simulink model "Integrate_SubMode_Motor_2021b"  (R2021b)
settings: Solver=FixedStepAuto  StartTime=0.0  StopTime=inf  FixedStep=Ts  RelTol=1e-3  EnableMultiTasking=on
values from neighbouring files (symbols this model uses):
  den_Gd = Gd.Den{:}    [para.m]
  Ki = 0.003    [para.m]
  Kp = 0.0001    [para.m]
  num_Gd = Gd.Num{:}    [para.m]
  rpm_scale = 1/12/4*60    (= 1.25)    [para.m]
  Ts = 0.01    [para.m]
  Wref = 4000    [para.m]
undefined symbols (not defined in the file or in its folder): ADC_MAX, cycle_per_rotate, ENCODER_MAX, Kd, RPM_MAX, sec_per_minute
libraries: arduinolib x17, simulink x4, arduinosensorlib x4, slpidlib x1
settings Model: SimulationMode=external  ExtModeTrigDuration=2  Creator=user  LastModifiedBy=user
settings SolverCC: AutoInsertRateTranBlk=on
settings OptimizationCC: EnhancedBackFolding=on  PassReuseOutputArgsAs=Individual arguments  ZeroExternalMemoryAtStartup=off  ZeroInternalMemoryAtStartup=off  MaxStackSize=64  OptimizeBlockOrder=speed  DifferentSizesBufferReuse=on  OptimizationCustomize=off  EfficientTunableParamExpr=on
settings DebuggingCC: ParameterTunabilityLossMsg=error
settings HardwareCC: ProdBitPerInt=16  ProdBitPerPointer=16  ProdBitPerSizeT=16  ProdBitPerPtrDiffT=16  ProdLargestAtomicFloat=None  ProdWordSize=8  ProdHWDeviceType=Atmel->AVR
settings SFSimCC: MATLABDynamicMemAlloc=off
settings RTWCC: Description=Embedded Coder  SystemTargetFile=ert.tlc  HardwareBoard=Arduino Mega 2560  TemplateMakefile=ert_default_tmf  Toolchain=Arduino AVR  BuildConfiguration=Faster Runs
settings CodeAppCC: ForceParamTrailComments=on  IgnoreCustomStorageClasses=off  OperatorAnnotations=on  SimulinkDataObjDesc=on  SFDataObjDesc=on  InsertBlockDesc=on
settings ERTTargetCC: SupportContinuousTime=on  SupportVariableSizeSignals=on  ExtMode=on  ExtModeStaticAlloc=on  ExtModeStaticAllocSize=2048  ExtModeMexArgs='' 0 17725

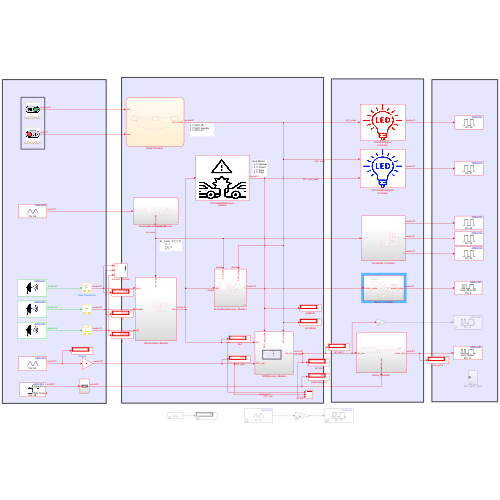
[thumbnail: Simulink's stored preview of the top-level diagram]
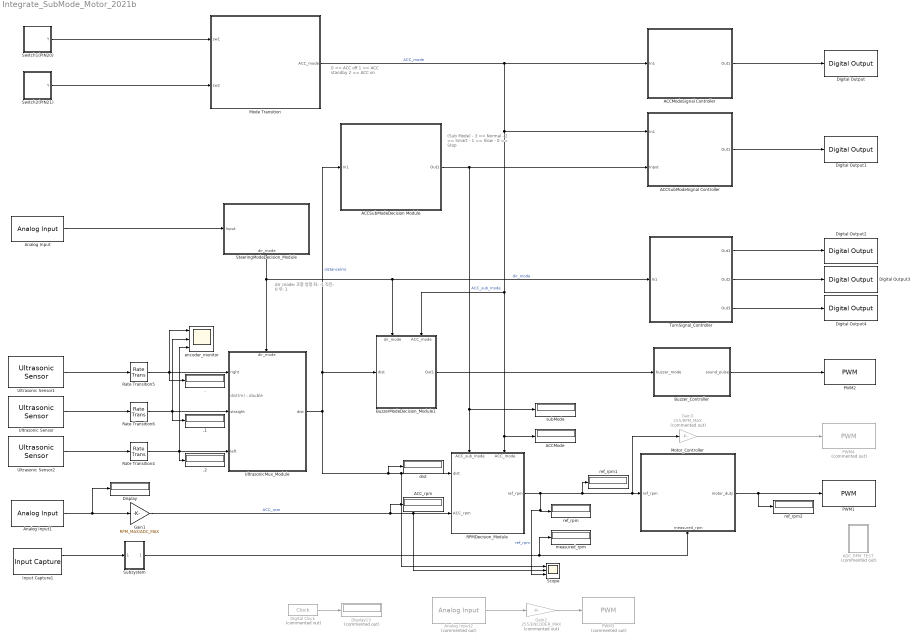
== system Integrate_SubMode_Motor_2021b ==
  note: dist(m) : double
  note: dir_mode: 조향 방향
      |  	좌: -1
      |  	직진: 0
      |  	우: 1
  note: 0 == ACC off
      | 1 == ACC standby
      | 2 == ACC on
  note: (Sub Mode)
      | - 3 == Normal
      | - 2 == Smart
      | - 1 == Slow
      | - 0 == Stop
  . : Display
  .1 : Display
  .2 : Display
  ACCMode : Display
  ACCModeSignal Controller : Subsystem
      mask Display: image('$imagefile'); % 변경하려면 툴스트립에 있는 "이미지 편집"을 사용하십시오.
  ACCSubModeDecision Module : Subsystem
      mask Display: image('$imagefile'); % 변경하려면 툴스트립에 있는 "이미지 편집"을 사용하십시오.
  ACCSubModeSignal Controller : Subsystem
      mask Display: image('$imagefile'); % 변경하려면 툴스트립에 있는 "이미지 편집"을 사용하십시오.
  ACC_rpm : Display
  ADC_RPM_TEST : Subsystem  Commented=on
  Analog Input : arduinolib/Analog Input  pinNumber=8  ReadResultsOnly=off  ConversionTriggerSource=Software  ExternalTriggerType=uint32( 0 )  OutputDataType=uint16  EnableConversionCompleteNotify=off  EnableOuputStatus=off  SampleTime=Ts  blockPlatform=arduino
  Analog Input1 : arduinolib/Analog Input  pinNumber=0  ReadResultsOnly=off  ConversionTriggerSource=Software  ExternalTriggerType=uint32( 0 )  OutputDataType=uint16  EnableConversionCompleteNotify=off  EnableOuputStatus=off  SampleTime=Ts  blockPlatform=arduino
  Analog Input2 : arduinolib/Analog Input  Commented=on  pinNumber=0  ReadResultsOnly=off  ConversionTriggerSource=Software  ExternalTriggerType=uint32( 0 )  OutputDataType=uint16  EnableConversionCompleteNotify=off  EnableOuputStatus=off  SampleTime=-1  blockPlatform=arduino
  BuzzerModeDecision_Module1 : Subsystem
      settings: PortSchema="{\"entries\":[{\"content\":{\"sides\":[{\"content\":{\"connectorIds\":[\"In1\"]},\"type\":\"ConnectorPlacement.EquallySpacedRectSide\",\"uuid\":\"3bfd8a6a-6750-43b9-a34d-1030ee4edf99\"},{\"content\":{\"connectorIds\":[\"Out1\"],\"side\":\"RIGHT\"},\"type\":\"ConnectorPlacement.EquallySpacedRectSide\",\"uuid\":\"183584f3-ff01-485d-aa62-5859e0907314\"},{\"content\":{\"connectorIds\":[\"In2\",\"In3\"],\"side\":\"TOP\"},\"type\":\"ConnectorPlacement.EquallySpacedRectSide\",\"uuid\":\"c1dfd82e-f053-4e34-bada-190db50d8d84\"}]},\"type\":\"ConnectorPlacement.EquallySpacedConnector\",\"uuid\":\"77a311fc-b440-4422-9bc9-ecab92f49ada\"}],\"packageUris\":[\"http://schema.mathworks.com/mf0/Connector/R2020b\"],\"version\":\"1.0\"}"
  Buzzer_Controller : Subsystem
  Digital Clock : DigitalClock  Commented=on
  Digital Output : arduinolib/Digital Output  pinNumber=30  Direction=output  blockPlatform=arduino
  Digital Output1 : arduinolib/Digital Output  pinNumber=31  Direction=output  blockPlatform=arduino
  Digital Output2 : arduinolib/Digital Output  pinNumber=44  Direction=output  blockPlatform=arduino
  Digital Output3 : arduinolib/Digital Output  pinNumber=45  Direction=output  blockPlatform=arduino
  Digital Output4 : arduinolib/Digital Output  pinNumber=46  Direction=output  blockPlatform=arduino
  Display : Display
  Display13 : Display  Commented=on
  Gain1 : Gain  Gain=RPM_MAX/ADC_MAX  OutDataTypeStr=double
  Gain2 : Gain  Commented=on  Gain=255/ENCODER_MAX  OutDataTypeStr=uint8
  Gain3 : Gain  Commented=on  Gain=255/RPM_MAX  OutDataTypeStr=uint8
  Input Capture1 : arduinolib/Input Capture  InputCapturePinNumber=48  SampleTime=Ts
      settings: SourceProductBaseCode=ARDUINO
  Mode Transition : Stateflow chart  TreatAsAtomicUnit=on
  "Motor_Controller " : Subsystem
      settings: PortSchema="{\"entries\":[{\"content\":{\"sides\":[{\"content\":{\"connectorIds\":[\"In1\"]},\"type\":\"ConnectorPlacement.EquallySpacedRectSide\",\"uuid\":\"84689b2b-9686-426f-98fe-832cf395d002\"},{\"content\":{\"connectorIds\":[\"Out1\"],\"side\":\"RIGHT\"},\"type\":\"ConnectorPlacement.EquallySpacedRectSide\",\"uuid\":\"269242fc-eb89-45a4-87bc-61aca4f4f947\"},{\"content\":{\"connectorIds\":[],\"side\":\"TOP\"},\"type\":\"ConnectorPlacement.EquallySpacedRectSide\",\"uuid\":\"b9328928-0765-4378-bf75-ce4fabb3519d\"},{\"content\":{\"connectorIds\":[\"In2\"],\"side\":\"BOTTOM\"},\"type\":\"ConnectorPlacement.EquallySpacedRectSide\",\"uuid\":\"a1cd2956-9074-43ce-a6b3-b2f914fe9274\"}]},\"type\":\"ConnectorPlacement.EquallySpacedConnector\",\"uuid\":\"faaddabd-e074-42ac-a65b-a2c01548f534\"}],\"packageUris\":[\"http://schema.mathworks.com/mf0/Connector/R2020b\"],\"version\":\"1.0\"}"
  PWM1 : arduinolib/PWM  pinNumber=11  frequencyType=Default  desiredFrequency=490.2  achievableFrequency=490.2
  PWM2 : arduinolib/PWM  pinNumber=5  frequencyType=Specify  desiredFrequency=490.2  achievableFrequency=490.1961
  PWM3 : arduinolib/PWM  Commented=on  pinNumber=11  frequencyType=Default  desiredFrequency=490.2  achievableFrequency=490.2
  PWM4 : arduinolib/PWM  Commented=on  pinNumber=11  frequencyType=Default  desiredFrequency=490.2  achievableFrequency=490.2
  RPMDecision_Module : Subsystem
      settings: PortSchema="{\"entries\":[{\"content\":{\"sides\":[{\"content\":{\"connectorIds\":[\"In1\",\"In2\"]},\"type\":\"ConnectorPlacement.EquallySpacedRectSide\",\"uuid\":\"6ec364ce-34b2-4beb-b97a-f32003c79d6e\"},{\"content\":{\"connectorIds\":[\"Out1\"],\"side\":\"RIGHT\"},\"type\":\"ConnectorPlacement.EquallySpacedRectSide\",\"uuid\":\"dc876503-cb4c-4ae1-9014-14ad87bdb333\"},{\"content\":{\"connectorIds\":[\"In3\",\"In4\"],\"side\":\"TOP\"},\"type\":\"ConnectorPlacement.EquallySpacedRectSide\",\"uuid\":\"5447802f-a25d-4c34-9dc6-d7b36056ed0d\"}]},\"type\":\"ConnectorPlacement.EquallySpacedConnector\",\"uuid\":\"292fcb4a-6f45-4a66-adbd-fd22b6096994\"}],\"packageUris\":[\"http://schema.mathworks.com/mf0/Connector/R2020b\"],\"version\":\"1.0\"}"
  Rate Transition4 : RateTransition  Deterministic=off  OutPortSampleTime=Ts
  Rate Transition5 : RateTransition  Deterministic=off  OutPortSampleTime=Ts
  Rate Transition6 : RateTransition  Deterministic=off  OutPortSampleTime=Ts
  Scope : Scope  NumInputPorts=3
  SteeringModeDecision_Module : Subsystem
      settings: PortSchema="{\"entries\":[{\"content\":{\"sides\":[{\"content\":{\"connectorIds\":[\"In1\"]},\"type\":\"ConnectorPlacement.EquallySpacedRectSide\",\"uuid\":\"81aef089-e139-4a21-a559-f4cfcbe1fd6b\"},{\"content\":{\"connectorIds\":[],\"side\":\"RIGHT\"},\"type\":\"ConnectorPlacement.EquallySpacedRectSide\",\"uuid\":\"59a5580f-3b8b-4c0e-b6d8-e62868ebf4fd\"},{\"content\":{\"connectorIds\":[],\"side\":\"TOP\"},\"type\":\"ConnectorPlacement.EquallySpacedRectSide\",\"uuid\":\"52e3278b-fe84-4ffc-bd60-3e79fa1021a4\"},{\"content\":{\"connectorIds\":[\"Out1\"],\"side\":\"BOTTOM\"},\"type\":\"ConnectorPlacement.EquallySpacedRectSide\",\"uuid\":\"1683fe8c-8f20-453b-887e-9deee14294f2\"}]},\"type\":\"ConnectorPlacement.EquallySpacedConnector\",\"uuid\":\"f0c787f9-8860-4fe5-8e2c-91ccd075b91e\"}],\"packageUris\":[\"http://schema.mathworks.com/mf0/Connector/R2020b\"],\"version\":\"1.0\"}"
  Subsystem : Subsystem
  Switch1(PIN20) : Subsystem
      mask Display: image('$imagefile'); % 변경하려면 툴스트립에 있는 "이미지 편집"을 사용하십시오.
  Switch2(PIN21) : Subsystem
      mask Display: image('$imagefile'); % 변경하려면 툴스트립에 있는 "이미지 편집"을 사용하십시오.
  TurnSignal_Controller : Subsystem
  Ultrasonic Sensor : arduinosensorlib/Ultrasonic Sensor  NumSignalPins=2  TrigPin=36  EchoPin=37  SignalPin=3  SampleTime_=0.3  blockPlatform=ARDUINO
      settings: SourceProductBaseCode=ARDUINO
  Ultrasonic Sensor1 : arduinosensorlib/Ultrasonic Sensor  NumSignalPins=2  TrigPin=38  EchoPin=39  SignalPin=3  SampleTime_=0.3  blockPlatform=ARDUINO
      settings: SourceProductBaseCode=ARDUINO
  Ultrasonic Sensor2 : arduinosensorlib/Ultrasonic Sensor  NumSignalPins=2  TrigPin=42  EchoPin=43  SignalPin=3  SampleTime_=0.3  blockPlatform=ARDUINO
      settings: SourceProductBaseCode=ARDUINO
  UltrasonicMux_Module : Subsystem
      settings: PortSchema="{\"entries\":[{\"content\":{\"sides\":[{\"content\":{\"connectorIds\":[\"In1\",\"In2\",\"In3\"]},\"type\":\"ConnectorPlacement.EquallySpacedRectSide\",\"uuid\":\"5f4ad8f0-04c3-4479-9dfd-33641402f242\"},{\"content\":{\"connectorIds\":[\"Out1\"],\"side\":\"RIGHT\"},\"type\":\"ConnectorPlacement.EquallySpacedRectSide\",\"uuid\":\"c4451af6-64c8-402e-8ffe-feeed5b209e6\"},{\"content\":{\"connectorIds\":[\"In4\"],\"side\":\"TOP\"},\"type\":\"ConnectorPlacement.EquallySpacedRectSide\",\"uuid\":\"4be8f8c7-8102-4379-8072-e8a8027f489d\"}]},\"type\":\"ConnectorPlacement.EquallySpacedConnector\",\"uuid\":\"2bd08bb9-e7f4-4004-b808-4b0f9daf5a96\"}],\"packageUris\":[\"http://schema.mathworks.com/mf0/Connector/R2020b\"],\"version\":\"1.0\"}"
  dist : Display
  encoder_monitor : Scope  NumInputPorts=3
  measured_rpm : Display
  ref_rpm : Display
  ref_rpm1 : Display
  ref_rpm2 : Display
  subMode : Display
  wires:
  Gain1/1 -> ACC_rpm/1, Scope/2, RPMDecision_Module/2(ACC_rpm)  "ACC_rpm"
  Ultrasonic Sensor2/1 -> Rate Transition4/1
  Analog Input1/1 -> Display/1, Gain1/1
  RPMDecision_Module/1(ref_rpm) -> ref_rpm1/1, "Motor_Controller "/1(ref_rpm), Gain3/1, Scope/3, ref_rpm/1  "ref_rpm"
  UltrasonicMux_Module/1(dist) -> dist/1, Scope/1, RPMDecision_Module/1(dist), ACCSubModeDecision Module/1(In1), BuzzerModeDecision_Module1/1(dist)  "distance(m)"
  Switch2(PIN21)/1(Y) -> Mode Transition/2(sw2)
  Switch1(PIN20)/1(Y) -> Mode Transition/1(sw1)
  Mode Transition/1(ACC_mode) -> ACCMode/1, RPMDecision_Module/4(ACC_mode), BuzzerModeDecision_Module1/3(ACC_mode), ACCSubModeSignal Controller/1(In1), ACCModeSignal Controller/1(In1)  "ACC_mode"
  ACCSubModeDecision Module/1(Out1) -> ACCSubModeSignal Controller/2(Input), RPMDecision_Module/3(ACC_sub_mode), subMode/1  "ACC_sub_mode"
  ACCModeSignal Controller/1(Out1) -> Digital Output/1
  ACCSubModeSignal Controller/1(Out1) -> Digital Output1/1
  Rate Transition4/1 -> .2/1, encoder_monitor/3, UltrasonicMux_Module/3(left)
  SteeringModeDecision_Module/1(dir_mode) -> TurnSignal_Controller/1(In1), BuzzerModeDecision_Module1/2(dir_mode), UltrasonicMux_Module/4(dir_mode)  "dir_mode"
  Buzzer_Controller/1(sound_pulse) -> PWM2/1
  TurnSignal_Controller/1(Out1) -> Digital Output2/1
  TurnSignal_Controller/2(Out2) -> Digital Output3/1
  TurnSignal_Controller/3(Out3) -> Digital Output4/1
  Analog Input/1 -> SteeringModeDecision_Module/1(Input)
  Ultrasonic Sensor/1 -> Rate Transition6/1
  Ultrasonic Sensor1/1 -> Rate Transition5/1
  Digital Clock/1 -> Display13/1
  BuzzerModeDecision_Module1/1(Out1) -> Buzzer_Controller/1(buzzer_mode)
  "Motor_Controller "/1(motor_duty) -> ref_rpm2/1, PWM1/1
  Rate Transition5/1 -> UltrasonicMux_Module/1(right), ./1, encoder_monitor/1
  Rate Transition6/1 -> .1/1, encoder_monitor/2, UltrasonicMux_Module/2(straight)
  Analog Input2/1 -> Gain2/1
  Gain2/1 -> PWM3/1
  Input Capture1/1 -> Subsystem/1(In1)
  Subsystem/1(measured_rpm) -> measured_rpm/1, "Motor_Controller "/2(measured_rpm)
  Gain3/1 -> PWM4/1

== system Integrate_SubMode_Motor_2021b/ACCModeSignal Controller ==
  In1 : Inport
  Constant : Constant
  If : If  IfExpression=u1==2  ElseIfExpressions=u1==1
  If Action Subsystem : Subsystem  TreatAsAtomicUnit=on
  If Action Subsystem2 : Subsystem  TreatAsAtomicUnit=on
  If Action Subsystem3 : Subsystem  TreatAsAtomicUnit=on
  Merge : Merge  Inputs=3
  Pulse Generator1 : DiscretePulseGenerator  PulseType=Time based  Period=1  PulseWidth=50  SampleTime=-1
  Pulse Generator3 : DiscretePulseGenerator  PulseType=Time based  Period=0.2  PulseWidth=50  SampleTime=-1
  Out1 : Outport
  wires:
  If Action Subsystem2/1(Out1) -> Merge/3
  Pulse Generator1/1 -> If Action Subsystem2/1(In1)
  Pulse Generator3/1 -> If Action Subsystem/1(In1)
  Merge/1 -> Out1/1
  If Action Subsystem/1(Out1) -> Merge/2
  If/1 -> If Action Subsystem3/Action
  If/2 -> If Action Subsystem/Action
  Constant/1 -> If Action Subsystem3/1(In1)
  If/3 -> If Action Subsystem2/Action
  If Action Subsystem3/1(Out1) -> Merge/1
  In1/1 -> If/1

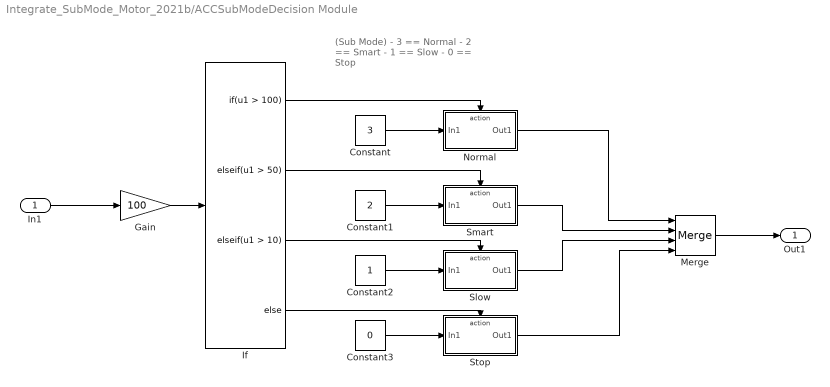
== system Integrate_SubMode_Motor_2021b/ACCSubModeDecision Module ==
  note: (Sub Mode)
      | - 3 == Normal
      | - 2 == Smart
      | - 1 == Slow
      | - 0 == Stop
  In1 : Inport
  Constant : Constant  Value=3
  Constant1 : Constant  Value=2
  Constant2 : Constant
  Constant3 : Constant  Value=0
  Gain : Gain  Gain=100
  If : If  IfExpression=u1 > 100  ElseIfExpressions=u1 > 50, u1 > 10
  Merge : Merge  Inputs=4
  "Normal " : Subsystem  TreatAsAtomicUnit=on
  Slow : Subsystem  TreatAsAtomicUnit=on
  Smart : Subsystem  TreatAsAtomicUnit=on
  Stop : Subsystem  TreatAsAtomicUnit=on
  Out1 : Outport
  wires:
  Slow/1(Out1) -> Merge/3
  Smart/1(Out1) -> Merge/2
  "Normal "/1(Out1) -> Merge/1
  Gain/1 -> If/1
  Constant2/1 -> Slow/1(In1)
  Constant/1 -> "Normal "/1(In1)
  In1/1 -> Gain/1
  Merge/1 -> Out1/1
  If/1 -> "Normal "/Action
  Constant3/1 -> Stop/1(In1)
  If/2 -> Smart/Action
  If/3 -> Slow/Action
  If/4 -> Stop/Action
  Stop/1(Out1) -> Merge/4
  Constant1/1 -> Smart/1(In1)

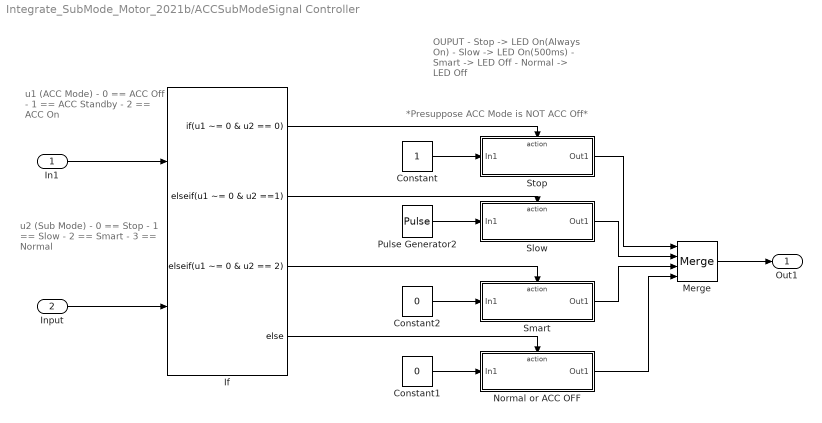
== system Integrate_SubMode_Motor_2021b/ACCSubModeSignal Controller ==
  note: u2 (Sub Mode)
      | - 0 == Stop
      | - 1 == Slow
      | - 2 == Smart
      | - 3 == Normal
  note: u1 (ACC Mode)
      | - 0 == ACC Off
      | - 1 == ACC Standby
      | - 2 ==  ACC On
  note: OUPUT
      | - Stop -> LED On(Always On)
      | - Slow -> LED On(500ms)
      | - Smart -> LED Off
      | - Normal -> LED Off
  note: *Presuppose ACC Mode is NOT ACC Off*
  In1 : Inport
  Input : Inport  Port=2
  Constant : Constant
  Constant1 : Constant  Value=0
  Constant2 : Constant  Value=0
  If : If  NumInputs=2  IfExpression=u1 ~= 0 & u2 == 0  ElseIfExpressions=u1 ~= 0 & u2 ==1, u1 ~= 0 & u2 == 2
  Merge : Merge  Inputs=4
  Normal or ACC OFF : Subsystem  TreatAsAtomicUnit=on
  Pulse Generator2 : DiscretePulseGenerator  PulseType=Time based  Period=0.2  PulseWidth=50  SampleTime=-1
  Slow : Subsystem  TreatAsAtomicUnit=on
  Smart : Subsystem  TreatAsAtomicUnit=on
  Stop : Subsystem  TreatAsAtomicUnit=on
  Out1 : Outport
  wires:
  Constant1/1 -> Normal or ACC OFF/1(In1)
  Pulse Generator2/1 -> Slow/1(In1)
  Merge/1 -> Out1/1
  Slow/1(Out1) -> Merge/2
  Constant/1 -> Stop/1(In1)
  Stop/1(Out1) -> Merge/1
  In1/1 -> If/1
  Input/1 -> If/2
  Constant2/1 -> Smart/1(In1)
  Normal or ACC OFF/1(Out1) -> Merge/4
  Smart/1(Out1) -> Merge/3
  If/1 -> Stop/Action
  If/2 -> Slow/Action
  If/3 -> Smart/Action
  If/4 -> Normal or ACC OFF/Action

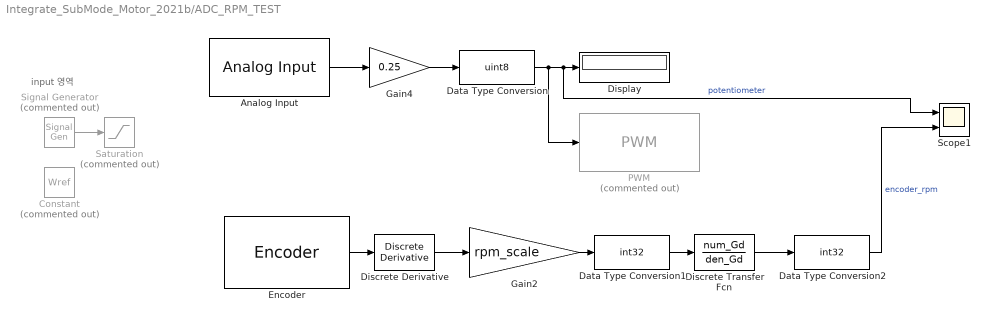
== system Integrate_SubMode_Motor_2021b/ADC_RPM_TEST ==
  note: input 영역
  Analog Input : arduinolib/Analog Input  pinNumber=0  ReadResultsOnly=off  ConversionTriggerSource=Software  ExternalTriggerType=uint32( 0 )  OutputDataType=uint16  EnableConversionCompleteNotify=off  EnableOuputStatus=off  SampleTime=-1  blockPlatform=arduino
  Constant : Constant  Commented=on  Value=Wref
  Data Type Conversion : DataTypeConversion  OutDataTypeStr=uint8
  Data Type Conversion1 : DataTypeConversion  OutDataTypeStr=int32
  Data Type Conversion2 : DataTypeConversion  OutDataTypeStr=int32
  Discrete Transfer Fcn : DiscreteTransferFcn  Numerator=num_Gd  Denominator=den_Gd
  Discrete Derivative : simulink/Discrete/Discrete Derivative  gainval=1.0  ICPrevScaledInput=0.0  OutMin=[]  OutMax=[]  OutDataType=fixdt(1, 16)  OutScaling=2^-10  DoSatur=off
  Display : Display
  Encoder : arduinosensorlib/Encoder  InputA=18  InputB=19  Mode=No reset  SampleTime=-1
      settings: SourceProductBaseCode=ARDUINO
  Gain2 : Gain  Gain=rpm_scale  OutDataTypeStr=double
  Gain4 : Gain  Gain=0.25
  PWM : arduinolib/PWM  Commented=on  pinNumber=11  frequencyType=Default  desiredFrequency=490.2  achievableFrequency=490.2
  Saturation : Saturate  Commented=on  UpperLimit=inf  LowerLimit=0
  Scope1 : Scope  NumInputPorts=2
  Signal Generator : SignalGenerator  Commented=on  Amplitude=5300  Frequency=0.1  Units=rad/sec
  wires:
  Discrete Transfer Fcn/1 -> Data Type Conversion2/1
  Encoder/1 -> Discrete Derivative/1
  Analog Input/1 -> Gain4/1
  Data Type Conversion1/1 -> Discrete Transfer Fcn/1
  Gain4/1 -> Data Type Conversion/1
  Data Type Conversion/1 -> PWM/1, Scope1/1, Display/1  "potentiometer"
  Discrete Derivative/1 -> Gain2/1
  Gain2/1 -> Data Type Conversion1/1
  Data Type Conversion2/1 -> Scope1/2  "encoder_rpm"
  Signal Generator/1 -> Saturation/1

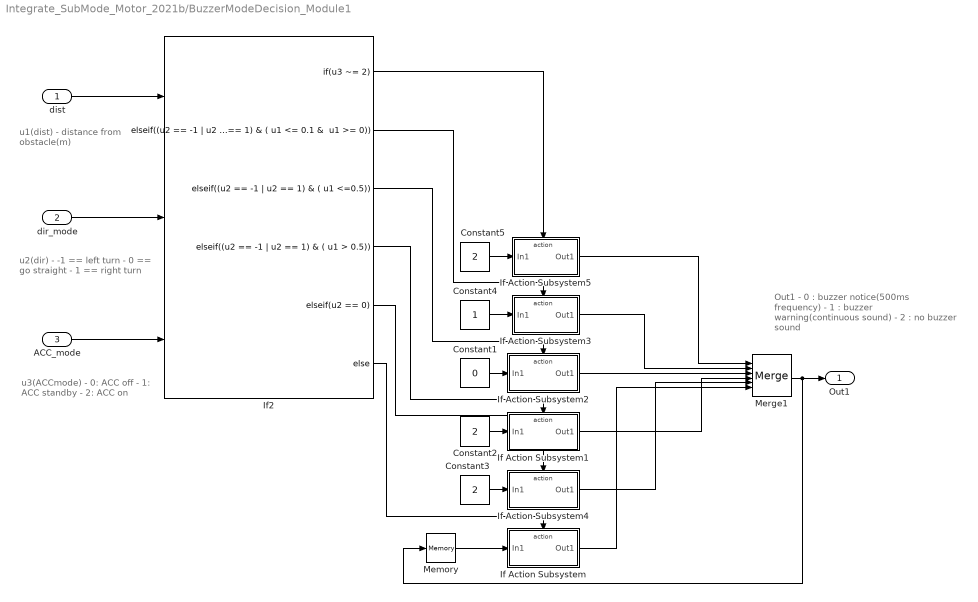
== system Integrate_SubMode_Motor_2021b/BuzzerModeDecision_Module1 ==
  note: u2(dir)
      | - -1 == left turn
      | - 0 == go straight
      | - 1 == right turn
  note: u1(dist)
      | - distance from obstacle(m)
  note: Out1
      | - 0 : buzzer notice(500ms frequency)
      | - 1 : buzzer warning(continuous sound)
      | - 2 : no buzzer sound
  note: u3(ACCmode)
      | - 0: ACC off
      | - 1: ACC standby
      | - 2: ACC on
  dist : Inport
  dir_mode : Inport  Port=2
  ACC_mode : Inport  Port=3  OutDataTypeStr=double
  Constant1 : Constant  Value=0
  Constant2 : Constant  Value=2
  Constant3 : Constant  Value=2
  Constant4 : Constant
  Constant5 : Constant  Value=2
  If Action Subsystem : Subsystem  TreatAsAtomicUnit=on
  If Action Subsystem1 : Subsystem  TreatAsAtomicUnit=on
  If Action Subsystem2 : Subsystem  TreatAsAtomicUnit=on
  If Action Subsystem3 : Subsystem  TreatAsAtomicUnit=on
  If Action Subsystem4 : Subsystem  TreatAsAtomicUnit=on
  If Action Subsystem5 : Subsystem  TreatAsAtomicUnit=on
  If2 : If  NumInputs=3  IfExpression=u3 ~= 2  ElseIfExpressions="(u2 == -1 | u2 == 1) & ( u1 <= 0.1 &  u1 >= 0), (u2 == -1 | u2 == 1) & ( u1 <=0.5) , (u2 == -1 | u2 == 1) & ( u1 > 0.5) ,  u2 == 0"
  Memory : Memory
  Merge1 : Merge  Inputs=6
  Out1 : Outport
  wires:
  If Action Subsystem/1(Out1) -> Merge1/6
  Memory/1 -> If Action Subsystem/1(In1)
  Constant4/1 -> If Action Subsystem3/1(In1)
  If Action Subsystem2/1(Out1) -> Merge1/3
  If Action Subsystem3/1(Out1) -> Merge1/2
  Constant1/1 -> If Action Subsystem2/1(In1)
  Constant2/1 -> If Action Subsystem1/1(In1)
  If Action Subsystem1/1(Out1) -> Merge1/4
  Constant3/1 -> If Action Subsystem4/1(In1)
  If Action Subsystem4/1(Out1) -> Merge1/5
  Merge1/1 -> Out1/1, Memory/1
  ACC_mode/1 -> If2/3
  If2/3 -> If Action Subsystem2/Action
  If2/2 -> If Action Subsystem3/Action
  If2/4 -> If Action Subsystem1/Action
  If2/5 -> If Action Subsystem4/Action
  If2/1 -> If Action Subsystem5/Action
  Constant5/1 -> If Action Subsystem5/1(In1)
  If Action Subsystem5/1(Out1) -> Merge1/1
  If2/6 -> If Action Subsystem/Action
  dir_mode/1 -> If2/2
  dist/1 -> If2/1

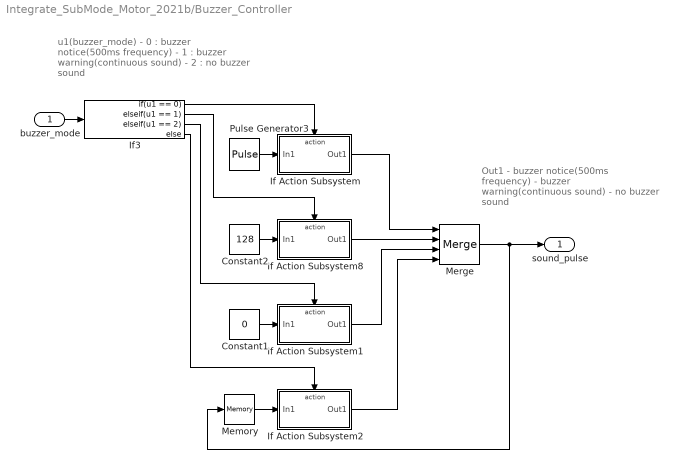
== system Integrate_SubMode_Motor_2021b/Buzzer_Controller ==
  note: u1(buzzer_mode)
      | - 0 : buzzer notice(500ms frequency)
      | - 1 : buzzer warning(continuous sound)
      | - 2 : no buzzer sound
  note: Out1
      | - buzzer notice(500ms frequency)
      | - buzzer warning(continuous sound)
      | - no buzzer sound
  buzzer_mode : Inport
  Constant1 : Constant  Value=0
  Constant2 : Constant  Value=128  OutDataTypeStr=double
  If Action Subsystem : Subsystem  TreatAsAtomicUnit=on
  If Action Subsystem1 : Subsystem  TreatAsAtomicUnit=on
  If Action Subsystem2 : Subsystem  TreatAsAtomicUnit=on
  If Action Subsystem8 : Subsystem  TreatAsAtomicUnit=on
  If3 : If  IfExpression=u1 == 0  ElseIfExpressions=u1 == 1, u1 == 2
  Memory : Memory
  Merge : Merge  Inputs=4
  Pulse Generator3 : DiscretePulseGenerator  PulseType=Time based  Amplitude=128  Period=0.5  PulseWidth=50
  sound_pulse : Outport
  wires:
  Constant1/1 -> If Action Subsystem1/1(In1)
  If Action Subsystem1/1(Out1) -> Merge/3
  Pulse Generator3/1 -> If Action Subsystem/1(In1)
  Merge/1 -> Memory/1, sound_pulse/1
  If3/2 -> If Action Subsystem8/Action
  Constant2/1 -> If Action Subsystem8/1(In1)
  If Action Subsystem/1(Out1) -> Merge/1
  buzzer_mode/1 -> If3/1
  If3/1 -> If Action Subsystem/Action
  Memory/1 -> If Action Subsystem2/1(In1)
  If3/4 -> If Action Subsystem2/Action
  If3/3 -> If Action Subsystem1/Action
  If Action Subsystem2/1(Out1) -> Merge/4
  If Action Subsystem8/1(Out1) -> Merge/2

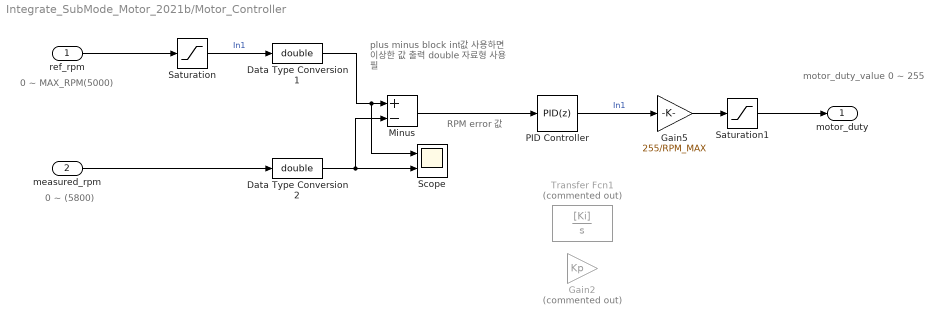
== system Integrate_SubMode_Motor_2021b/Motor_Controller  ==
  note: RPM error 값
  note: 0 ~ MAX_RPM(5000)
  note: motor_duty_value
      | 0 ~ 255
  note: 0 ~ (5800)
  note: plus minus block
      | int값 사용하면 이상한 값 출력
      | double 자료형 사용 필
  ref_rpm : Inport
  measured_rpm : Inport  Port=2
  Data Type Conversion1 : DataTypeConversion  OutDataTypeStr=double
  Data Type Conversion2 : DataTypeConversion  OutDataTypeStr=double
  Gain2 : Gain  Commented=on  Gain=Kp  OutDataTypeStr=double
  Gain5 : Gain  Gain=255/RPM_MAX
  Minus : Sum  Inputs=+-
  PID Controller : slpidlib/PID Controller  Controller=PID  Form=Parallel  TimeDomain=Discrete-time  UseExternalTs=off  SampleTime=-1  IntegratorMethod=Forward Euler  FilterMethod=Forward Euler  ControllerParametersSource=internal  P=Kp  I=Ki  D=Kd  UseFilter=on  N=100  TunerSelectOption=Transfer Function Based (PID Tuner App)  InitialConditionSource=internal  InitialConditionForIntegrator=0  InitialConditionForFilter=0  DifferentiatorICPrevScaledInput=0  ExternalReset=none  TrackingMode=off  Kt=1  LimitOutput=on  SatLimitsSource=internal  UpperSaturationLimit=inf  LowerSaturationLimit=0  LinearizeAsGain=on  AntiWindupMode=back-calculation  Kb=1  POutMin=[]  POutMax=[]  IOutMin=[]  IOutMax=[]  DOutMin=[]  DOutMax=[]  NOutMin=[]  NOutMax=[]  SumOutMin=[]  SumOutMax=[]  SaturationOutMin=[]  SaturationOutMax=[]  PParamMin=[]  PParamMax=[]  IParamMin=[]  IParamMax=[]  DParamMin=[]  DParamMax=[]  NParamMin=[]  NParamMax=[]  KbParamMin=[]  KbParamMax=[]  KtParamMin=[]  KtParamMax=[]  KbOutMin=[]  KbOutMax=[]  KtOutMin=[]  KtOutMax=[]  IntegratorOutMin=[]  IntegratorOutMax=[]  FilterOutMin=[]  FilterOutMax=[]  SumI1OutMin=[]  SumI1OutMax=[]  SumI2OutMin=[]  SumI2OutMax=[]  SumI3OutMin=[]  SumI3OutMax=[]  SumI4OutMin=[]  SumI4OutMax=[]  SumDOutMin=[]  SumDOutMax=[]  DifferentiatorOutMin=[]  DifferentiatorOutMax=[]  FilterDiffOutCoefMin=[]  FilterDiffOutCoefMax=[]  ReciprocalOutMin=[]  ReciprocalOutMax=[]  SumDenOutMin=[]  SumDenOutMax=[]  SumNumOutMin=[]  SumNumOutMax=[]  DivideOutMin=[]  DivideOutMax=[]  UdiffTsProdOutMin=[]  UdiffTsProdOutMax=[]  NTsProdOutMin=[]  NTsProdOutMax=[]  UintegralTsProdOutMin=[]  UintegralTsProdOutMax=[]  UngainTsProdOutMin=[]  UngainTsProdOutMax=[]  FilterDenConstantOutDataTypeStr=Inherit: Inherit via back propagation  FilterDenConstantOutMin=[]  FilterDenConstantOutMax=[]  PCopyOutDataTypeStr=Inherit: Inherit via back propagation  PCopyOutMin=[]  PCopyOutMax=[]  NCopyOutDataTypeStr=Inherit: Inherit via back propagation  NCopyOutMin=[]  NCopyOutMax=[]  IntegratorContinuousStateAttributes=''  IntegratorStateMustResolveToSignalObject=off  IntegratorRTWStateStorageClass=Auto  FilterContinuousStateAttributes=''  FilterStateMustResolveToSignalObject=off  FilterRTWStateStorageClass=Auto  ParallelPVariant=InternalParameters  IdealPVariant=Disabled  IVariant=InternalParameters  DVariant=InternalParameters  IntegratorVariant=Discrete  SatVariant=Enabled  AWVariant=BackCalculation  PCopyVariant=Disabled  TRVariant=Disabled  FdbkBlocksVariant=Forward  IdealPFdbkVariant=Disabled  SatFdbkVariant=Disabled  DerivativeFilterVariant=ForwardEulerFilter  NVariant=InternalParameters  NCopyVariant=Disabled  FilterICVariant=InternalICsFilter  IntegratorICVariant=InternalICs  ExternalResetVariant=Disabled  TRSumVariant=Passthrough  SumFdbkVariant=Disabled  SumVariant=Sum_PID  TsampFilterVariant=InternalTs  TsampNgainVariant=Passthrough  TsampIntegralVariant=Passthrough  ExternalSaturationOutDataTypeStr=Inherit: Same as second input
  Saturation : Saturate  UpperLimit=RPM_MAX  LowerLimit=0
  Saturation1 : Saturate  UpperLimit=255  LowerLimit=0  OutDataTypeStr=uint8
  Scope : Scope  NumInputPorts=2
  Transfer Fcn1 : TransferFcn  Commented=on  Numerator=[Ki]  Denominator=[1 0]
  motor_duty : Outport
  wires:
  Gain5/1 -> Saturation1/1
  measured_rpm/1 -> Data Type Conversion2/1
  PID Controller/1 -> Gain5/1  "In1"
  ref_rpm/1 -> Saturation/1
  Saturation1/1 -> motor_duty/1
  Saturation/1 -> Data Type Conversion1/1  "In1"
  Data Type Conversion1/1 -> Scope/1, Minus/1
  Data Type Conversion2/1 -> Scope/2, Minus/2
  Minus/1 -> PID Controller/1

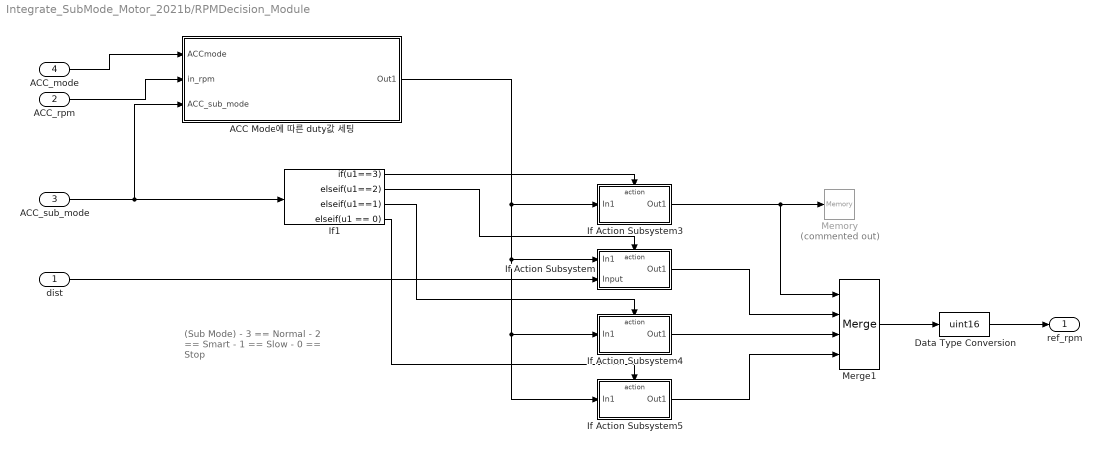
== system Integrate_SubMode_Motor_2021b/RPMDecision_Module ==
  note: (Sub Mode)
      | - 3 == Normal
      | - 2 == Smart
      | - 1 == Slow
      | - 0 == Stop
  dist : Inport
  ACC_rpm : Inport  Port=2
  ACC_sub_mode : Inport  Port=3
  ACC_mode : Inport  Port=4
  ACC Mode에 따른 duty값 세팅 : Subsystem
  Data Type Conversion : DataTypeConversion  OutDataTypeStr=uint16
  If Action Subsystem : Subsystem  TreatAsAtomicUnit=on
  If Action Subsystem3 : Subsystem  TreatAsAtomicUnit=on
  If Action Subsystem4 : Subsystem  TreatAsAtomicUnit=on
  If Action Subsystem5 : Subsystem  TreatAsAtomicUnit=on
  If1 : If  IfExpression=u1==3  ElseIfExpressions=u1==2, u1==1, u1 == 0  ShowElse=off
  Memory : Memory  Commented=on
  Merge1 : Merge  Inputs=4
  ref_rpm : Outport
  wires:
  ACC_sub_mode/1 -> ACC Mode에 따른 duty값 세팅/3(ACC_sub_mode), If1/1
  If Action Subsystem3/1(Out1) -> Memory/1, Merge1/1
  ACC Mode에 따른 duty값 세팅/1(Out1) -> If Action Subsystem5/1(In1), If Action Subsystem4/1(In1), If Action Subsystem/1(In1), If Action Subsystem3/1(In1)
  ACC_mode/1 -> ACC Mode에 따른 duty값 세팅/1(ACCmode)
  Merge1/1 -> Data Type Conversion/1
  dist/1 -> If Action Subsystem/2(Input)
  If Action Subsystem/1(Out1) -> Merge1/2
  If Action Subsystem4/1(Out1) -> Merge1/3
  If Action Subsystem5/1(Out1) -> Merge1/4
  If1/1 -> If Action Subsystem3/Action
  If1/2 -> If Action Subsystem/Action
  If1/3 -> If Action Subsystem4/Action
  If1/4 -> If Action Subsystem5/Action
  ACC_rpm/1 -> ACC Mode에 따른 duty값 세팅/2(in_rpm)
  Data Type Conversion/1 -> ref_rpm/1

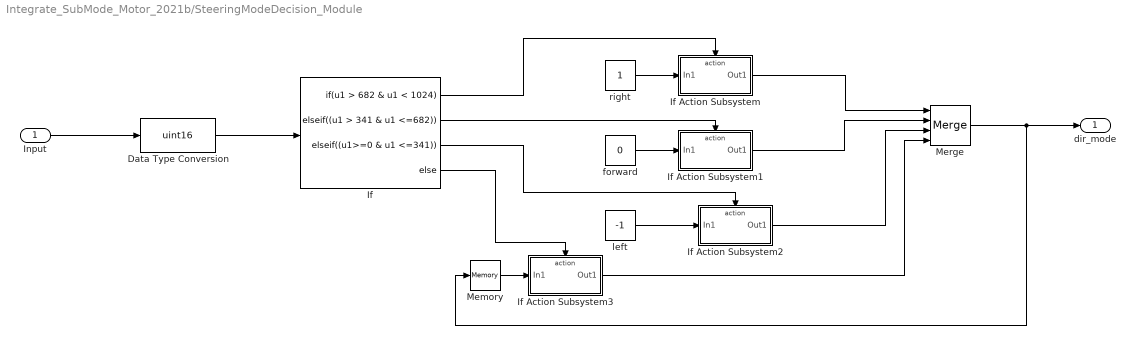
== system Integrate_SubMode_Motor_2021b/SteeringModeDecision_Module ==
  Input : Inport
  Data Type Conversion : DataTypeConversion  OutDataTypeStr=uint16
  If : If  IfExpression=u1 > 682 & u1 < 1024  ElseIfExpressions=(u1 > 341 & u1 <=682),(u1>=0 & u1 <=341)
  If Action Subsystem : Subsystem  TreatAsAtomicUnit=on
  If Action Subsystem1 : Subsystem  TreatAsAtomicUnit=on
  If Action Subsystem2 : Subsystem  TreatAsAtomicUnit=on
  If Action Subsystem3 : Subsystem  TreatAsAtomicUnit=on
  Memory : Memory
  Merge : Merge  Inputs=4
  forward : Constant  Value=0  OutDataTypeStr=double
  left : Constant  Value=-1  OutDataTypeStr=double
  right : Constant  OutDataTypeStr=double
  dir_mode : Outport
  wires:
  If Action Subsystem2/1(Out1) -> Merge/3
  If/1 -> If Action Subsystem/Action
  left/1 -> If Action Subsystem2/1(In1)
  forward/1 -> If Action Subsystem1/1(In1)
  If/2 -> If Action Subsystem1/Action
  If Action Subsystem/1(Out1) -> Merge/1
  If Action Subsystem1/1(Out1) -> Merge/2
  right/1 -> If Action Subsystem/1(In1)
  Merge/1 -> Memory/1, dir_mode/1
  Input/1 -> Data Type Conversion/1
  Data Type Conversion/1 -> If/1
  If/3 -> If Action Subsystem2/Action
  If/4 -> If Action Subsystem3/Action
  Memory/1 -> If Action Subsystem3/1(In1)
  If Action Subsystem3/1(Out1) -> Merge/4

== system Integrate_SubMode_Motor_2021b/Subsystem ==
  note: input
      | processing
  In1 : Inport
  Data Type Conversion1 : DataTypeConversion  OutDataTypeStr=uint16
  Gain2 : Gain  Gain=sec_per_minute/cycle_per_rotate  OutDataTypeStr=int32
  LPF difference : Scope  NumInputPorts=3
  Low-pass-filter : Subsystem
  my FIR : Subsystem
  measured_rpm : Outport
  wires:
  In1/1 -> Gain2/1, LPF difference/1
  Low-pass-filter/1(measured_rpm_f) -> Data Type Conversion1/1, LPF difference/3
  my FIR/1(y) -> Low-pass-filter/1(measured_rpm), LPF difference/2
  Data Type Conversion1/1 -> measured_rpm/1
  Gain2/1 -> my FIR/1(In1)

== system Integrate_SubMode_Motor_2021b/Switch1(PIN20) ==
  Detect Increase : simulink/Logic and Bit Operations/Detect Increase  vinit=0.0  OutDataTypeStr=boolean
  External Interrupt : arduinolib/External Interrupt  Pin=20  PullUp=on  Mode=FALLING  InterruptSimulationInput=off
      settings: SourceProductBaseCode=ARDUINO
  Function-Call Subsystem : Subsystem  TreatAsAtomicUnit=on
  Rate Transition : RateTransition  Integrity=off  Deterministic=off  OutPortSampleTime=Ts
  Y : Outport
  wires:
  Function-Call Subsystem/1(y) -> Rate Transition/1
  Rate Transition/1 -> Detect Increase/1
  External Interrupt/1 -> Function-Call Subsystem/Trigger
  Detect Increase/1 -> Y/1

== system Integrate_SubMode_Motor_2021b/Switch2(PIN21) ==
  Detect Increase1 : simulink/Logic and Bit Operations/Detect Increase  vinit=0.0  OutDataTypeStr=uint8
  External Interrupt1 : arduinolib/External Interrupt  Pin=21  PullUp=on  Mode=FALLING  InterruptSimulationInput=off
      settings: SourceProductBaseCode=ARDUINO
  Function-Call Subsystem1 : Subsystem  TreatAsAtomicUnit=on
  Rate Transition1 : RateTransition  Deterministic=off  OutPortSampleTime=Ts
  Y : Outport
  wires:
  Function-Call Subsystem1/1(Out1) -> Rate Transition1/1
  Rate Transition1/1 -> Detect Increase1/1
  External Interrupt1/1 -> Function-Call Subsystem1/Trigger
  Detect Increase1/1 -> Y/1

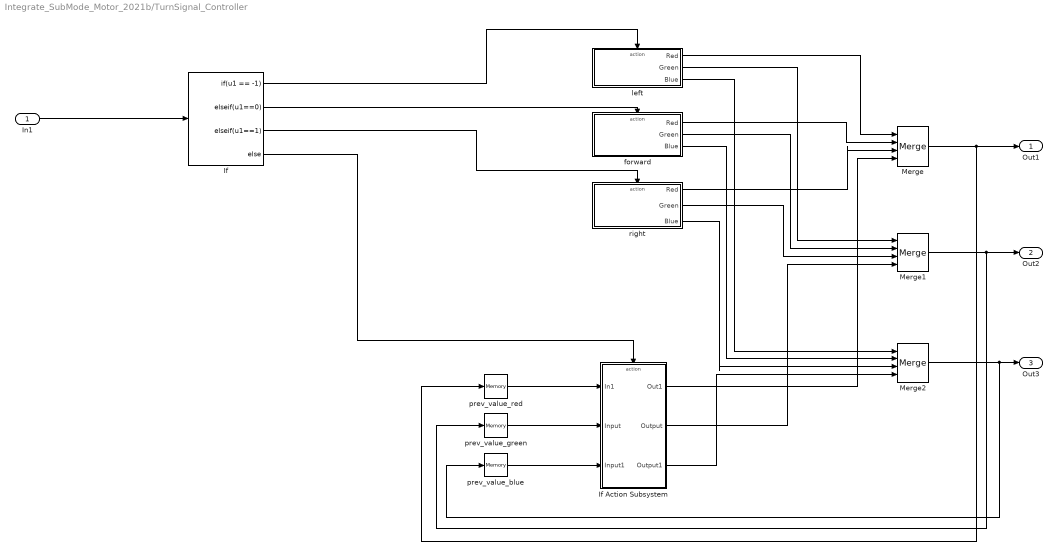
== system Integrate_SubMode_Motor_2021b/TurnSignal_Controller ==
  In1 : Inport
  If : If  IfExpression=u1 == -1  ElseIfExpressions=u1==0, u1==1
  If Action Subsystem : Subsystem  TreatAsAtomicUnit=on
  Merge : Merge  Inputs=4
  Merge1 : Merge  Inputs=4
  Merge2 : Merge  Inputs=4
  forward : Subsystem  TreatAsAtomicUnit=on
  left : Subsystem  TreatAsAtomicUnit=on
  prev_value_blue : Memory  InheritSampleTime=on
  prev_value_green : Memory  InheritSampleTime=on
  prev_value_red : Memory  InheritSampleTime=on
  right : Subsystem  TreatAsAtomicUnit=on
  Out1 : Outport
  Out2 : Outport  Port=2
  Out3 : Outport  Port=3
  wires:
  forward/3(Blue) -> Merge2/2
  In1/1 -> If/1
  right/2(Green) -> Merge1/3
  If/2 -> forward/Action
  prev_value_blue/1 -> If Action Subsystem/3(Input1)
  right/1(Red) -> Merge/3
  right/3(Blue) -> Merge2/3
  If/4 -> If Action Subsystem/Action
  forward/1(Red) -> Merge/2
  left/2(Green) -> Merge1/1
  forward/2(Green) -> Merge1/2
  If Action Subsystem/1(Out1) -> Merge/4
  Merge/1 -> Out1/1, prev_value_red/1
  Merge2/1 -> Out3/1, prev_value_blue/1
  left/1(Red) -> Merge/1
  If/3 -> right/Action
  Merge1/1 -> Out2/1, prev_value_green/1
  prev_value_green/1 -> If Action Subsystem/2(Input)
  prev_value_red/1 -> If Action Subsystem/1(In1)
  left/3(Blue) -> Merge2/1
  If Action Subsystem/3(Output1) -> Merge2/4
  If/1 -> left/Action
  If Action Subsystem/2(Output) -> Merge1/4

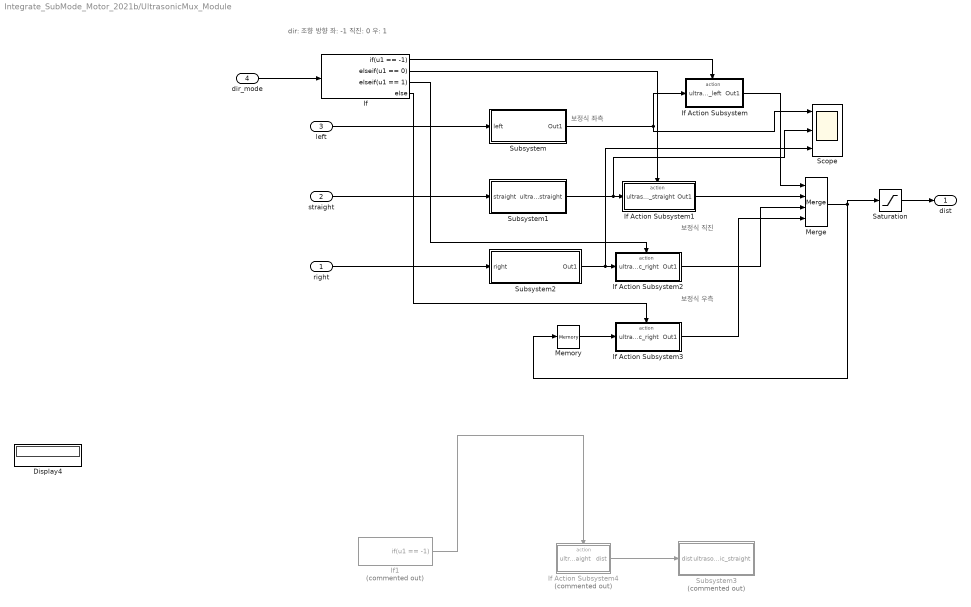
== system Integrate_SubMode_Motor_2021b/UltrasonicMux_Module ==
  note: 보정식 직진
  note: 보정식 좌측
  note: dir: 조향 방향
      |  	좌: -1
      |  	직진: 0
      |  	우: 1
  note: 보정식 우측
  right : Inport
  straight : Inport  Port=2
  left : Inport  Port=3
  dir_mode : Inport  Port=4
  Display4 : Display
  If : If  IfExpression=u1 == -1  ElseIfExpressions=u1 == 0, u1 == 1
  If Action Subsystem : Subsystem  TreatAsAtomicUnit=on
  If Action Subsystem1 : Subsystem  TreatAsAtomicUnit=on
  If Action Subsystem2 : Subsystem  TreatAsAtomicUnit=on
  If Action Subsystem3 : Subsystem  TreatAsAtomicUnit=on
  If Action Subsystem4 : Subsystem  Commented=on  TreatAsAtomicUnit=on
  If1 : If  Commented=on  IfExpression=u1 == -1  ShowElse=off
  Memory : Memory
  Merge : Merge  Inputs=4
  Saturation : Saturate  UpperLimit=2.3  LowerLimit=0
  Scope : Scope  NumInputPorts=3
  Subsystem : Subsystem
  Subsystem1 : Subsystem
  Subsystem2 : Subsystem
  Subsystem3 : Subsystem  Commented=on
  dist : Outport
  wires:
  If/1 -> If Action Subsystem/Action
  If/2 -> If Action Subsystem1/Action
  If Action Subsystem/1(Out1) -> Merge/1
  Merge/1 -> Saturation/1, Memory/1
  Subsystem/1(Out1) -> If Action Subsystem/1(ultrasonic_left), Scope/1
  Subsystem1/1(ultrasonic_straight) -> Scope/2, If Action Subsystem1/1(ultrasonic_straight)
  If Action Subsystem1/1(Out1) -> Merge/2
  If Action Subsystem2/1(Out1) -> Merge/3
  Subsystem2/1(Out1) -> Scope/3, If Action Subsystem2/1(ultrasonic_right)
  If/3 -> If Action Subsystem2/Action
  Memory/1 -> If Action Subsystem3/1(ultrasonic_right)
  If/4 -> If Action Subsystem3/Action
  If Action Subsystem3/1(Out1) -> Merge/4
  If Action Subsystem4/1(dist) -> Subsystem3/1(dist)
  If1/1 -> If Action Subsystem4/Action
  Saturation/1 -> dist/1
  right/1 -> Subsystem2/1(right)
  dir_mode/1 -> If/1
  left/1 -> Subsystem/1(left)
  straight/1 -> Subsystem1/1(straight)

== system Integrate_SubMode_Motor_2021b/ACCModeSignal Controller/If Action Subsystem ==
  In1 : Inport
  Action Port : ActionPort  ActionPortLabel=elseif(u1==1)
  Out1 : Outport
  wires:
  In1/1 -> Out1/1

== system Integrate_SubMode_Motor_2021b/ACCModeSignal Controller/If Action Subsystem2 ==
  In1 : Inport
  Action Port : ActionPort  ActionPortLabel=else
  Out1 : Outport
  wires:
  In1/1 -> Out1/1

== system Integrate_SubMode_Motor_2021b/ACCModeSignal Controller/If Action Subsystem3 ==
  In1 : Inport
  Action Port : ActionPort  ActionPortLabel=if(u1==2)
  Out1 : Outport
  wires:
  In1/1 -> Out1/1

== system Integrate_SubMode_Motor_2021b/ACCSubModeDecision Module/Normal  ==
  In1 : Inport
  Action Port : ActionPort  ActionPortLabel=if(u1 > 100)
  Out1 : Outport
  wires:
  In1/1 -> Out1/1

== system Integrate_SubMode_Motor_2021b/ACCSubModeDecision Module/Slow ==
  In1 : Inport
  Action Port : ActionPort  ActionPortLabel=elseif( u1 > 10)
  Out1 : Outport
  wires:
  In1/1 -> Out1/1

== system Integrate_SubMode_Motor_2021b/ACCSubModeDecision Module/Smart ==
  In1 : Inport
  Action Port : ActionPort  ActionPortLabel=elseif(u1 > 50)
  Out1 : Outport
  wires:
  In1/1 -> Out1/1

== system Integrate_SubMode_Motor_2021b/ACCSubModeDecision Module/Stop ==
  In1 : Inport
  Action Port : ActionPort  ActionPortLabel=else
  Out1 : Outport
  wires:
  In1/1 -> Out1/1

== system Integrate_SubMode_Motor_2021b/ACCSubModeSignal Controller/Normal or ACC OFF ==
  In1 : Inport
  Action Port : ActionPort  ActionPortLabel=else
  Out1 : Outport
  wires:
  In1/1 -> Out1/1

== system Integrate_SubMode_Motor_2021b/ACCSubModeSignal Controller/Slow ==
  In1 : Inport
  Action Port : ActionPort  ActionPortLabel=elseif(u1 ~= 0 & u2 ==1)
  Out1 : Outport
  wires:
  In1/1 -> Out1/1

== system Integrate_SubMode_Motor_2021b/ACCSubModeSignal Controller/Smart ==
  In1 : Inport
  Action Port : ActionPort  ActionPortLabel=elseif( u1 ~= 0 & u2 == 2)
  Out1 : Outport
  wires:
  In1/1 -> Out1/1

== system Integrate_SubMode_Motor_2021b/ACCSubModeSignal Controller/Stop ==
  In1 : Inport
  Action Port : ActionPort  ActionPortLabel=if(u1 ~= 0 & u2 == 0)
  Out1 : Outport
  wires:
  In1/1 -> Out1/1

== system Integrate_SubMode_Motor_2021b/BuzzerModeDecision_Module1/If Action Subsystem ==
  In1 : Inport
  Action Port : ActionPort  ActionPortLabel=else
  Out1 : Outport
  wires:
  In1/1 -> Out1/1

== system Integrate_SubMode_Motor_2021b/BuzzerModeDecision_Module1/If Action Subsystem1 ==
  In1 : Inport
  Action Port : ActionPort  ActionPortLabel=elseif( (u2 == -1 | u2 == 1) & ( u1 > 0.5) )
  Out1 : Outport
  wires:
  In1/1 -> Out1/1

== system Integrate_SubMode_Motor_2021b/BuzzerModeDecision_Module1/If Action Subsystem2 ==
  In1 : Inport
  Action Port : ActionPort  ActionPortLabel=elseif( (u2 == -1 | u2 == 1) & ( u1 <=0.5) )
  Out1 : Outport
  wires:
  In1/1 -> Out1/1

== system Integrate_SubMode_Motor_2021b/BuzzerModeDecision_Module1/If Action Subsystem3 ==
  In1 : Inport
  Action Port : ActionPort  ActionPortLabel="elseif((u2 == -1 | u2 == 1) & ( u1 <= 0.1 &  u1 >= 0))"
  Out1 : Outport
  wires:
  In1/1 -> Out1/1

== system Integrate_SubMode_Motor_2021b/BuzzerModeDecision_Module1/If Action Subsystem4 ==
  In1 : Inport
  Action Port : ActionPort  ActionPortLabel="elseif(  u2 == 0)"
  Out1 : Outport
  wires:
  In1/1 -> Out1/1

== system Integrate_SubMode_Motor_2021b/BuzzerModeDecision_Module1/If Action Subsystem5 ==
  In1 : Inport
  Action Port : ActionPort  ActionPortLabel=if(u3 ~= 2)
  Out1 : Outport
  wires:
  In1/1 -> Out1/1

== system Integrate_SubMode_Motor_2021b/Buzzer_Controller/If Action Subsystem ==
  In1 : Inport
  Action Port : ActionPort  ActionPortLabel=if(u1 == 0)
  Out1 : Outport
  wires:
  In1/1 -> Out1/1

== system Integrate_SubMode_Motor_2021b/Buzzer_Controller/If Action Subsystem1 ==
  In1 : Inport
  Action Port : ActionPort  ActionPortLabel=elseif( u1 == 2)
  Out1 : Outport  LockScale=on
  wires:
  In1/1 -> Out1/1

== system Integrate_SubMode_Motor_2021b/Buzzer_Controller/If Action Subsystem2 ==
  In1 : Inport
  Action Port : ActionPort  ActionPortLabel=else
  Out1 : Outport
  wires:
  In1/1 -> Out1/1

== system Integrate_SubMode_Motor_2021b/Buzzer_Controller/If Action Subsystem8 ==
  In1 : Inport
  Action Port : ActionPort  ActionPortLabel=elseif(u1 == 1)
  Out1 : Outport
  wires:
  In1/1 -> Out1/1

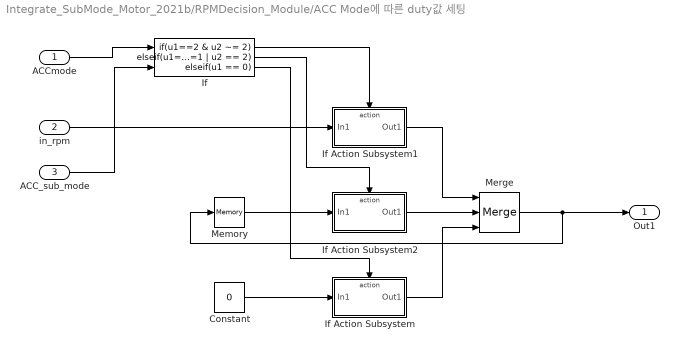
== system Integrate_SubMode_Motor_2021b/RPMDecision_Module/ACC Mode에 따른 duty값 세팅 ==
  ACCmode : Inport
  in_rpm : Inport  Port=2
  ACC_sub_mode : Inport  Port=3
  Constant : Constant  Value=0  OutDataTypeStr=double
  If : If  NumInputs=2  IfExpression=u1==2 & u2 ~= 2  ElseIfExpressions=u1==1 | u2 == 2, u1 == 0  ShowElse=off
  If Action Subsystem : Subsystem  TreatAsAtomicUnit=on
  If Action Subsystem1 : Subsystem  TreatAsAtomicUnit=on
  If Action Subsystem2 : Subsystem  TreatAsAtomicUnit=on
  Memory : Memory
  Merge : Merge  Inputs=3
  Out1 : Outport
  wires:
  Constant/1 -> If Action Subsystem/1(In1)
  in_rpm/1 -> If Action Subsystem1/1(In1)
  If/2 -> If Action Subsystem2/Action
  If/3 -> If Action Subsystem/Action
  Memory/1 -> If Action Subsystem2/1(In1)
  Merge/1 -> Out1/1, Memory/1
  If/1 -> If Action Subsystem1/Action
  If Action Subsystem1/1(Out1) -> Merge/1
  If Action Subsystem2/1(Out1) -> Merge/2
  If Action Subsystem/1(Out1) -> Merge/3
  ACCmode/1 -> If/1
  ACC_sub_mode/1 -> If/2

== system Integrate_SubMode_Motor_2021b/RPMDecision_Module/If Action Subsystem ==
  In1 : Inport
  Input : Inport  Port=2
  Action Port : ActionPort  ActionPortLabel=elseif(u1==2)
  Product : Product
  Out1 : Outport
  wires:
  In1/1 -> Product/1
  Input/1 -> Product/2
  Product/1 -> Out1/1

== system Integrate_SubMode_Motor_2021b/RPMDecision_Module/If Action Subsystem3 ==
  In1 : Inport
  Action Port : ActionPort  ActionPortLabel=if(u1==3)
  Out1 : Outport  OutDataTypeStr=double
  wires:
  In1/1 -> Out1/1

== system Integrate_SubMode_Motor_2021b/RPMDecision_Module/If Action Subsystem4 ==
  In1 : Inport
  Action Port : ActionPort  ActionPortLabel=elseif( u1==1)
  Gain : Gain  Gain=0.5  OutDataTypeStr=double
  Out1 : Outport  OutDataTypeStr=double
  wires:
  In1/1 -> Gain/1
  Gain/1 -> Out1/1

== system Integrate_SubMode_Motor_2021b/RPMDecision_Module/If Action Subsystem5 ==
  In1 : Inport
  Action Port : ActionPort  ActionPortLabel=elseif( u1 == 0)
  Gain : Gain  Gain=0  OutDataTypeStr=double
  Out1 : Outport
  wires:
  In1/1 -> Gain/1
  Gain/1 -> Out1/1

== system Integrate_SubMode_Motor_2021b/SteeringModeDecision_Module/If Action Subsystem ==
  In1 : Inport
  Action Port : ActionPort  ActionPortLabel=if(u1 > 682 & u1 < 1024)
  Out1 : Outport
  wires:
  In1/1 -> Out1/1

== system Integrate_SubMode_Motor_2021b/SteeringModeDecision_Module/If Action Subsystem1 ==
  In1 : Inport
  Action Port : ActionPort  ActionPortLabel=elseif((u1 > 341 & u1 <=682))
  Out1 : Outport
  wires:
  In1/1 -> Out1/1

== system Integrate_SubMode_Motor_2021b/SteeringModeDecision_Module/If Action Subsystem2 ==
  In1 : Inport
  Action Port : ActionPort  ActionPortLabel=elseif((u1>=0 & u1 <=341))
  Out1 : Outport
  wires:
  In1/1 -> Out1/1

== system Integrate_SubMode_Motor_2021b/SteeringModeDecision_Module/If Action Subsystem3 ==
  In1 : Inport
  Action Port : ActionPort  ActionPortLabel=else
  Out1 : Outport
  wires:
  In1/1 -> Out1/1

== system Integrate_SubMode_Motor_2021b/Subsystem/Low-pass-filter ==
  measured_rpm : Inport
  Data Type Conversion2 : DataTypeConversion  OutDataTypeStr=int32
  Discrete Transfer Fcn : DiscreteTransferFcn  Numerator=num_Gd  Denominator=den_Gd
  Gain3 : Gain  Commented=on  Gain=60/(2*pi)  OutDataTypeStr=double
  Scope : Scope  NumInputPorts=2
  Scope1 : Scope  Commented=on
  rpm : Display  Commented=on
  type conversion(rpm) : Display
  measured_rpm_f : Outport
  wires:
  Gain3/1 -> rpm/1, Scope1/1
  measured_rpm/1 -> Gain3/1, Scope/2, type conversion(rpm)/1, Discrete Transfer Fcn/1
  Discrete Transfer Fcn/1 -> Data Type Conversion2/1
  Data Type Conversion2/1 -> Scope/1, measured_rpm_f/1

== system Integrate_SubMode_Motor_2021b/Subsystem/my FIR ==
  In1 : Inport
  Constant2 : Constant  Value=300
  Memory : Memory
  Minus : Sum  Inputs=+-
  Plus : Sum
  Saturation Dynamic : simulink/Discontinuities/Saturation Dynamic  OutMin=[]  OutMax=[]  OutDataTypeStr=Inherit: Same as second input  OutDataType=fixdt(1, 16)  OutScaling=2^-10  DoSatur=off
  y : Outport
  wires:
  In1/1 -> Saturation Dynamic/2
  Memory/1 -> Minus/1, Plus/1
  Saturation Dynamic/1 -> y/1, Memory/1
  Minus/1 -> Saturation Dynamic/3
  Constant2/1 -> Minus/2, Plus/2
  Plus/1 -> Saturation Dynamic/1

== system Integrate_SubMode_Motor_2021b/Switch1(PIN20)/Function-Call Subsystem ==
  function : TriggerPort  TriggerType=function-call  VariantControl=(inherit)
  Constant : Constant
  Sum : Sum  Inputs=|++
  Unit Delay : UnitDelay  SampleTime=-1  HasFrameUpgradeWarning=on
  y : Outport
  wires:
  Unit Delay/1 -> Sum/2
  Constant/1 -> Sum/1
  Sum/1 -> Unit Delay/1, y/1

== system Integrate_SubMode_Motor_2021b/Switch2(PIN21)/Function-Call Subsystem1 ==
  function : TriggerPort  TriggerType=function-call  VariantControl=(inherit)
  Constant : Constant
  Sum : Sum  Inputs=|++
  Unit Delay : UnitDelay  SampleTime=-1  HasFrameUpgradeWarning=on
  Out1 : Outport
  wires:
  Sum/1 -> Unit Delay/1, Out1/1
  Unit Delay/1 -> Sum/2
  Constant/1 -> Sum/1

== system Integrate_SubMode_Motor_2021b/TurnSignal_Controller/If Action Subsystem ==
  In1 : Inport
  Input : Inport  Port=2
  Input1 : Inport  Port=3
  Action Port : ActionPort  ActionPortLabel=else
  Out1 : Outport
  Output : Outport  Port=2
  Output1 : Outport  Port=3
  wires:
  In1/1 -> Out1/1
  Input/1 -> Output/1
  Input1/1 -> Output1/1

== system Integrate_SubMode_Motor_2021b/TurnSignal_Controller/forward ==
  Action Port : ActionPort  ActionPortLabel=elseif(u1==0)
  Constant : Constant  Value=0
  Constant1 : Constant
  Constant2 : Constant  Value=0
  Red : Outport
  Green : Outport  Port=2
  Blue : Outport  Port=3
  wires:
  Constant2/1 -> Blue/1
  Constant1/1 -> Green/1
  Constant/1 -> Red/1

== system Integrate_SubMode_Motor_2021b/TurnSignal_Controller/left ==
  Action Port : ActionPort  ActionPortLabel=if(u1 == -1)
  Constant : Constant  Value=0
  Constant1 : Constant  Value=0
  Pulse Generator : DiscretePulseGenerator  Period=20  PulseWidth=10  SampleTime=-1
  Red : Outport
  Green : Outport  Port=2
  Blue : Outport  Port=3
  wires:
  Pulse Generator/1 -> Red/1
  Constant/1 -> Green/1
  Constant1/1 -> Blue/1

== system Integrate_SubMode_Motor_2021b/TurnSignal_Controller/right ==
  Action Port : ActionPort  ActionPortLabel=elseif( u1==1)
  Constant : Constant  Value=0
  Constant1 : Constant  Value=0
  Pulse Generator : DiscretePulseGenerator  Period=20  PulseWidth=10  SampleTime=-1
  Red : Outport
  Green : Outport  Port=2
  Blue : Outport  Port=3
  wires:
  Constant1/1 -> Red/1
  Pulse Generator/1 -> Blue/1
  Constant/1 -> Green/1

== system Integrate_SubMode_Motor_2021b/UltrasonicMux_Module/If Action Subsystem ==
  ultrasonic_left : Inport
  Action Port : ActionPort  ActionPortLabel=if(u1 == -1)
  Out1 : Outport
  wires:
  ultrasonic_left/1 -> Out1/1

== system Integrate_SubMode_Motor_2021b/UltrasonicMux_Module/If Action Subsystem1 ==
  ultrasonic_straight : Inport
  Action Port : ActionPort  ActionPortLabel=elseif(u1 == 0)
  Out1 : Outport
  wires:
  ultrasonic_straight/1 -> Out1/1

== system Integrate_SubMode_Motor_2021b/UltrasonicMux_Module/If Action Subsystem2 ==
  ultrasonic_right : Inport
  Action Port : ActionPort  ActionPortLabel=elseif( u1 == 1)
  Out1 : Outport
  wires:
  ultrasonic_right/1 -> Out1/1

== system Integrate_SubMode_Motor_2021b/UltrasonicMux_Module/If Action Subsystem3 ==
  ultrasonic_right : Inport
  Action Port : ActionPort  ActionPortLabel=else
  Out1 : Outport
  wires:
  ultrasonic_right/1 -> Out1/1

== system Integrate_SubMode_Motor_2021b/UltrasonicMux_Module/If Action Subsystem4 ==
  ultrasonic_straight : Inport
  Action Port : ActionPort  ActionPortLabel=if(u1 == -1)
  dist : Outport
  wires:
  ultrasonic_straight/1 -> dist/1

== system Integrate_SubMode_Motor_2021b/UltrasonicMux_Module/Subsystem ==
  note: y=1.0448x−0.4715
  left : Inport
  Constant : Constant  Value=0.4715
  Gain : Gain  Gain=1.0448
  Gain1 : Gain  Gain=100
  Gain2 : Gain  Gain=0.01
  Subtract : Sum  Inputs=+-
  Out1 : Outport
  wires:
  left/1 -> Gain1/1
  Gain/1 -> Subtract/1
  Constant/1 -> Subtract/2
  Gain1/1 -> Gain/1
  Subtract/1 -> Gain2/1
  Gain2/1 -> Out1/1

== system Integrate_SubMode_Motor_2021b/UltrasonicMux_Module/Subsystem1 ==
  note: y=1.0250x−0.2872
  straight : Inport
  Constant : Constant  Value=0.2872
  Gain : Gain  Gain=1.025
  Gain1 : Gain  Gain=100
  Gain2 : Gain  Gain=0.01
  Subtract : Sum  Inputs=+-
  ultrasonic_straight : Outport
  wires:
  Gain/1 -> Subtract/1
  Constant/1 -> Subtract/2
  straight/1 -> Gain1/1
  Gain1/1 -> Gain/1
  Gain2/1 -> ultrasonic_straight/1
  Subtract/1 -> Gain2/1

== system Integrate_SubMode_Motor_2021b/UltrasonicMux_Module/Subsystem2 ==
  note: y=1.01365272x−0.77147476
  right : Inport
  Constant : Constant  Value=0.771474
  Gain : Gain  Gain=1.013652
  Gain1 : Gain  Gain=100
  Gain2 : Gain  Gain=0.01
  Subtract : Sum  Inputs=+-
  Out1 : Outport
  wires:
  Gain/1 -> Subtract/1
  Constant/1 -> Subtract/2
  right/1 -> Gain1/1
  Subtract/1 -> Gain2/1
  Gain1/1 -> Gain/1
  Gain2/1 -> Out1/1

== system Integrate_SubMode_Motor_2021b/UltrasonicMux_Module/Subsystem3 ==
  note: y=1.0250x−0.2872
  dist : Inport
  Constant : Constant  Value=0.2872
  Gain : Gain  Gain=1.025
  Gain1 : Gain  Gain=100
  Gain2 : Gain  Gain=0.01
  Subtract : Sum  Inputs=+-
  ultrasonic_straight : Outport
  wires:
  Gain/1 -> Subtract/1
  Constant/1 -> Subtract/2
  dist/1 -> Gain1/1
  Gain1/1 -> Gain/1
  Gain2/1 -> ultrasonic_straight/1
  Subtract/1 -> Gain2/1

== system Integrate_SubMode_Motor_2021b/RPMDecision_Module/ACC Mode에 따른 duty값 세팅/If Action Subsystem ==
  In1 : Inport
  Action Port : ActionPort  ActionPortLabel=elseif( u1 == 0)
  Out1 : Outport
  wires:
  In1/1 -> Out1/1

== system Integrate_SubMode_Motor_2021b/RPMDecision_Module/ACC Mode에 따른 duty값 세팅/If Action Subsystem1 ==
  In1 : Inport
  Action Port : ActionPort  ActionPortLabel=if(u1==2 & u2 ~= 2)
  Out1 : Outport
  wires:
  In1/1 -> Out1/1

== system Integrate_SubMode_Motor_2021b/RPMDecision_Module/ACC Mode에 따른 duty값 세팅/If Action Subsystem2 ==
  In1 : Inport
  Action Port : ActionPort  ActionPortLabel=elseif(u1==1 | u2 == 2)
  Out1 : Outport
  wires:
  In1/1 -> Out1/1

== stateflow chart Integrate_SubMode_Motor_2021b/Mode Transition ==
  state ACC_off
    ACC_mode=0;
  state ACC_standby
    ACC_mode=1;
  state ACC_active
    ACC_mode=2;
  (default) -> ACC_off
  ACC_standby -> ACC_active [order 2] : [sw1==1 ]
  ACC_off -> ACC_standby : [sw1==1 ]
  ACC_standby -> ACC_off [order 1] : [sw2==1]
  ACC_active -> ACC_off : [sw1 == 1 || sw2 ==1]
  data: ACC_mode output; sw1 input; sw2 input
